simulink model "MBD_WEEK2_QN1"  (R2020b)
settings: Solver=VariableStepAuto  StartTime=0.0  StopTime=50  RelTol=1e-3
settings Model: Creator=dell  LastModifiedBy=dell

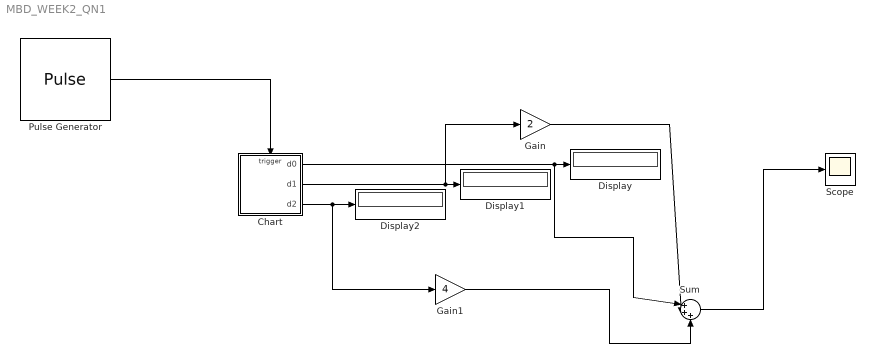
== system MBD_WEEK2_QN1 ==
  Chart : Stateflow chart  TreatAsAtomicUnit=on
  Display : Display
  Display1 : Display
  Display2 : Display
  Gain : Gain  Gain=2
  Gain1 : Gain  Gain=4
  Pulse Generator : DiscretePulseGenerator  PulseType=Time based  Period=1  PulseWidth=5
  Scope : Scope
  Sum : Sum  Inputs=|+++
  wires:
  Chart/1(d0) -> Sum/1, Display/1
  Chart/2(d1) -> Gain/1, Display1/1
  Chart/3(d2) -> Gain1/1, Display2/1
  Pulse Generator/1 -> Chart/Trigger
  Gain1/1 -> Sum/3
  Gain/1 -> Sum/2
  Sum/1 -> Scope/1

== stateflow chart MBD_WEEK2_QN1/Chart ==
  state Digit0 [parallel]
    settings: executionOrder=3
    state zero
      entry:
      d0=0;
    state one
      entry:
      d0=1;
    (default) -> Digit0.zero
    Digit0.zero -> Digit0.one : [reset==0]
    Digit0.one -> Digit0.zero : inputclick{inc2}
  state Digit1 [parallel]
    settings: executionOrder=2
    state zero
      entry:
      d1=0;
    state one
      entry:
      d1=1;
    (default) -> Digit1.zero
    Digit1.zero -> Digit1.one : inc2
    Digit1.one -> Digit1.zero : inc2{inc3}
  state Digit2 [parallel]
    settings: executionOrder=1
    state zero
      entry:
      d2=0;
      during:
      reset=0;
    state one
      entry:
      d2=1;
      reset=1;
    (default) -> Digit2.zero
    Digit2.zero -> Digit2.one : inc3
    Digit2.one -> Digit2.zero : inputclick
  data: d0 output; d1 output; d2 output; reset local
  events: inputclick input RISING_EDGE_EVENT; inc2 local RISING_EDGE_EVENT; inc3 local RISING_EDGE_EVENT
